simulink model "che322tutorial5"  (R2017a)
settings: Solver=ode4  StartTime=0.0  StopTime=10.0  FixedStep=0.01  RelTol=1e-3
settings Model: Creator=majeedhu  LastModifiedBy=donaghy1

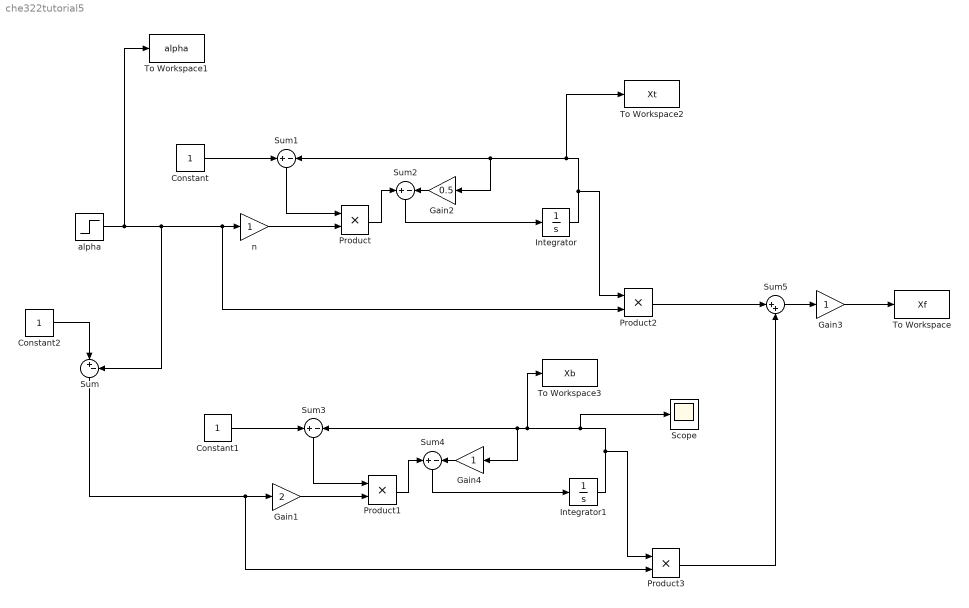
== system che322tutorial5 ==
  Constant : Constant
  Constant1 : Constant
  Constant2 : Constant
  Gain1 : Gain  Gain=2
  Gain2 : Gain  Gain=0.5
  Gain3 : Gain
  Gain4 : Gain
  Integrator : Integrator  InitialCondition=0.5
  Integrator1 : Integrator  InitialCondition=0.5
  Product{,1..3} (4 alike) : Product
  Scope : Scope
  Sum : Sum  Inputs=|+-
  Sum{1..4} (4 alike) : Sum  Inputs=+-
  Sum5 : Sum  Inputs=|++
  To Workspace : ToWorkspace  VariableName=Xf  SampleTime=-1
  To Workspace1 : ToWorkspace  VariableName=alpha  SampleTime=-1
  To Workspace2 : ToWorkspace  VariableName=Xt  SampleTime=-1
  To Workspace3 : ToWorkspace  VariableName=Xb  SampleTime=-1
  alpha : Step  Before=0.5  After=0.45  SampleTime=0
  n : Gain
  wires:
  Constant2/1 -> Sum/1
  alpha/1 -> To Workspace1/1, Product2/2, n/1, Sum/2
  Sum/1 -> Product3/2, Gain1/1
  Constant/1 -> Sum1/1
  Integrator/1 -> Product2/1, To Workspace2/1, Gain2/1, Sum1/2
  n/1 -> Product/2
  Sum1/1 -> Product/1
  Gain2/1 -> Sum2/2
  Product/1 -> Sum2/1
  Sum2/1 -> Integrator/1
  Integrator1/1 -> Product3/1, Scope/1, To Workspace3/1, Gain4/1, Sum3/2
  Product1/1 -> Sum4/1
  Sum3/1 -> Product1/1
  Sum4/1 -> Integrator1/1
  Gain4/1 -> Sum4/2
  Constant1/1 -> Sum3/1
  Gain1/1 -> Product1/2
  Product3/1 -> Sum5/2
  Product2/1 -> Sum5/1
  Sum5/1 -> Gain3/1
  Gain3/1 -> To Workspace/1
